simulink model "test1"  (R2020a)
settings: Solver=VariableStepAuto  StartTime=0.0  StopTime=inf  FixedStep=Ts  RelTol=1e-3
PostLoadFcn:
  | , if any(exist('dsrtsu_mdlpostloadfcn', 'file') ~= 0), dsrtsu_mdlpostloadfcn('Execute', bdroot); end,
InitFcn:
  | , if any(exist('rtifpga_mdlclblib', 'file') ~= 0), rtifpga_mdlclblib('Init', bdroot); end,
model workspace (MAT data in the model file):
  FPGA_test1_1_Interrupt_1_1_write = Simulink.Signal
  FPGA_test1_1_Interrupt_1_1_write.Description = 'RTIFPGA'
  FPGA_test1_1_Interrupt_1_1_write.DataType = 'double'
  FPGA_test1_1_Interrupt_1_1_write.Dimensions = '1'
  FPGA_test1_1_Interrupt_1_1_write.DimensionsMode = 'auto'
  FPGA_test1_1_Interrupt_1_1_write.Complexity = 'auto'
  FPGA_test1_1_Interrupt_1_1_write.SampleTime = -1
  FPGA_test1_1_Interrupt_1_1_write.SamplingMode = 'auto'
  FPGA_test1_1_Register_1_1_1_write = Simulink.Signal
  FPGA_test1_1_Register_1_1_1_write.Description = 'RTIFPGA'
  FPGA_test1_1_Register_1_1_1_write.DataType = 'double'
  FPGA_test1_1_Register_1_1_1_write.Dimensions = '1'
  FPGA_test1_1_Register_1_1_1_write.DimensionsMode = 'auto'
  FPGA_test1_1_Register_1_1_1_write.Complexity = 'auto'
  FPGA_test1_1_Register_1_1_1_write.SampleTime = -1
  FPGA_test1_1_Register_1_1_1_write.SamplingMode = 'auto'
  FPGA_test1_1_Register_2_1_1_write = Simulink.Signal
  FPGA_test1_1_Register_2_1_1_write.Description = 'RTIFPGA'
  FPGA_test1_1_Register_2_1_1_write.DataType = 'double'
  FPGA_test1_1_Register_2_1_1_write.Dimensions = '1'
  FPGA_test1_1_Register_2_1_1_write.DimensionsMode = 'auto'
  FPGA_test1_1_Register_2_1_1_write.Complexity = 'auto'
  FPGA_test1_1_Register_2_1_1_write.SampleTime = -1
  FPGA_test1_1_Register_2_1_1_write.SamplingMode = 'auto'
  FPGA_test1_1_Register_3_1_1_write = Simulink.Signal
  FPGA_test1_1_Register_3_1_1_write.Description = 'RTIFPGA'
  FPGA_test1_1_Register_3_1_1_write.DataType = 'double'
  FPGA_test1_1_Register_3_1_1_write.Dimensions = '1'
  FPGA_test1_1_Register_3_1_1_write.DimensionsMode = 'auto'
  FPGA_test1_1_Register_3_1_1_write.Complexity = 'auto'
  FPGA_test1_1_Register_3_1_1_write.SampleTime = -1
  FPGA_test1_1_Register_3_1_1_write.SamplingMode = 'auto'
  FPGA_test1_1_Register_4_1_1_write = Simulink.Signal
  FPGA_test1_1_Register_4_1_1_write.Description = 'RTIFPGA'
  FPGA_test1_1_Register_4_1_1_write.DataType = 'double'
  FPGA_test1_1_Register_4_1_1_write.Dimensions = '1'
  FPGA_test1_1_Register_4_1_1_write.DimensionsMode = 'auto'
  FPGA_test1_1_Register_4_1_1_write.Complexity = 'auto'
  FPGA_test1_1_Register_4_1_1_write.SampleTime = -1
  FPGA_test1_1_Register_4_1_1_write.SamplingMode = 'auto'
values from neighbouring files (symbols this model uses):
  clamp_threshold = 200    [param.m]
  io_fixed_gain = 10*1000/(3*100)    (= 33.3333333333)    [param.m]
  io_sonda_gain = 10/0.010    (= 1000)    [param.m]
  ioa_gain = 1    [param.m]
  ioa_offset = 0.12    [param.m]
  iob_gain = 1    [param.m]
  iob_offset = 0.06    [param.m]
  ioc_gain = 1    [param.m]
  ioc_offset = -0.1    [param.m]
  Ts = 20e-6    (= 2e-05)    [param.m]
  vclamp_gain = 1010    [param.m]
  vclamp_offset = 10.5    [param.m]
  vi_fixed_gain = 10*44    (= 440)    [param.m]
  vi_sonda_gain = 10*200    (= 2000)    [param.m]
  via_gain = 1    [param.m]
  via_offset = 2.2    [param.m]
  vib_gain = 1    [param.m]
  vib_offset = 3    [param.m]
  vic_gain = 1    [param.m]
  vic_offset = 4.2    [param.m]
libraries: xbsIndex_r4 x428, rti1202lib_adc_class1 x9, rtiproclib x6, simulink x2, rtifpgainterfacelib x1
(part 1 of 7)
Description:
  | Standard RTI1202 template.
  | Supported MATLAB version:  R2020a.
settings Model: Tag=RTI1202  DSRTSU_INTERNAL_RTI_VER=570  DSRTSU_INTERNAL_RTI_TYPE=rti1202  RTICANMMDATA=struct('GeneralSetupData',struct('modelroot','D:\MarcosGomez\test1','generalsettings',struct('filesettings',struct('destfolder',struct('Name','RTICANMM_FILES','Check',1),'buildfolder',struct('Name','.','Check',1),'AbsDestfolder',struct('Name','D:\MarcosGomez\test1\RTICANMM_FILES'),'AbsBuildfolder',struct('Name','D:\MarcosGomez\test1'))),'options',struct('addpaths',1,'rmpaths',1,'addtrcexclusion',true,'cannavigator',struct('checkmonitoring',0),'show_usrtrc',0,'use_usrtrc',0),'advanced',struct('options',ones(1,100)),'MPSetup',{{}},'RTI',struct('Type','RTI1202','Ver','7.15','Date','02-Nov-2020'),'modelname','test1','block','test1'))  DSRTSU_INTERNAL_RTIFPGA=170  OrderedModelArguments=off  Creator=dSPACE2020b  LastModifiedBy=dspace
settings DataIOCC: ReturnWorkspaceOutputs=off
settings OptimizationCC: BlockReduction=off  OptimizeBlockIOStorage=off  BufferReuse=off  GlobalBufferReuse=off  ExpressionFolding=off  LocalBlockOutputs=off  OptimizeDataStoreBuffers=off  BusAssignmentInplaceUpdate=off
settings DebuggingCC: PregeneratedLibrarySubsystemCodeDiagnostic=none  ArithmeticOperatorsInVariantConditions=warning
settings HardwareCC: ProdBitPerPointer=32  ProdBitPerSizeT=32  ProdBitPerPtrDiffT=32  ProdLargestAtomicInteger=Integer  ProdEndianess=BigEndian  ProdWordSize=32  ProdLongLongMode=on  ProdHWDeviceType=Custom Processor->Custom  TargetIntDivRoundTo=Zero  TargetEndianess=BigEndian  TargetHWDeviceType=Custom Processor->Custom
settings ModelReferenceCC: EnableParallelModelReferenceBuilds=on  ParallelModelReferenceMATLABWorkerInit=Load Top Model
settings SFSimCC: SimUseLocalCustomCode=off  MATLABDynamicMemAlloc=off  CustomCodeUndefinedFunction=UseInterfaceOnly
settings RTWCC: Description=dSPACE DS1202 Hardware Platform  SystemTargetFile=rti1202.tlc  MakeCommand=make_rti  TemplateMakefile=rti1202.tmf  RTWUseLocalCustomCode=off
settings CodeAppCC: StateflowObjectComments=on
settings STFCustomTargetCC: ParMdlRefBuildCompliant=on  SystemTargetFile=rti1202.tlc
settings GRTTargetCC: TargetLangStandard=C89/C90 (ANSI)  CompOptLevelCompliant=off  ConcurrentExecutionCompliant=off  CombineOutputUpdateFcns=off  MatFileLogging=off  CPPClassGenCompliant=off  UseToolchainInfoCompliant=off
settings ConfigComp: CovMetricSettings=dswe

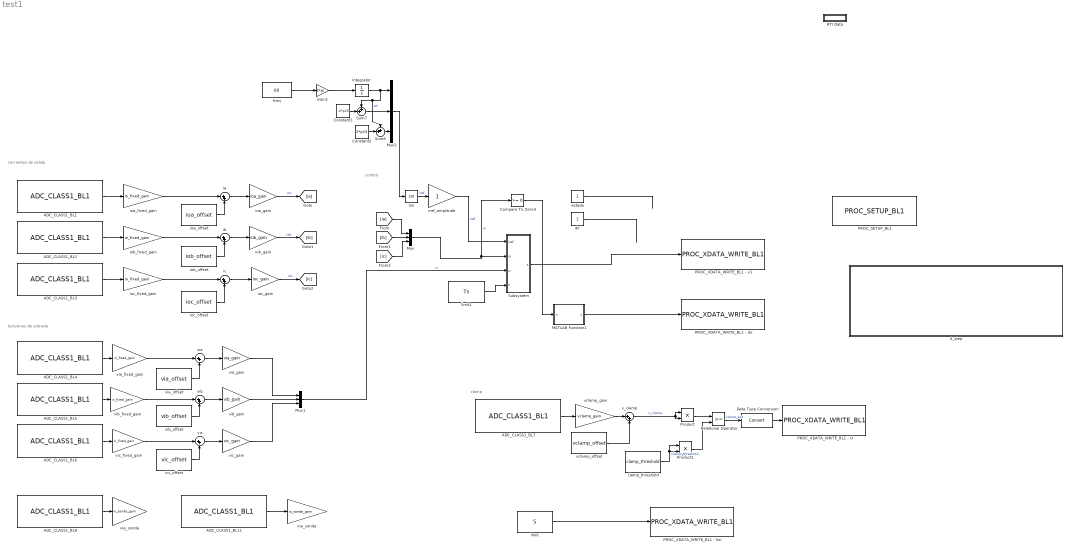
== system test1 ==
  note: control
  note: clamp
  note: tensiones de entrada
  note: corrientes de salida
  4_step : Subsystem
  ADC_CLASS1_BL1 : rti1202lib_adc_class1/ADC_CLASS1_BL1  DSProperties=struct('RTI',struct('Version',uint32(1),'BlockType',struct('isSLSource',uint8(1),'isSLSink',uint8(1),'isHWSource',uint8(0),'isHWSink',uint8(1),'isSetup',uint8(0),'isInline',uint8(1),'isNonInline',uint8(0),'isInterrupt',uint8(0),'isChannelwise',uint8(1)),'IOBoardType',{{'DS120X','STD','ADCC1'}},'UnitType','ADC','Identifier','ADC','DialogType','ML','BlockSet','NONE','SlaveProcessor','NONE'))  RTIBlockInterface=struct('InputPortsActive',0,'InputPortsWidth',int32(1),'InputPortsDataType',{{'SS_BOOLEAN'}},'InputPortsName',{{'Continue'}},'OutputPortsActive',[1 0],'OutputPortsWidth',int32([1 1]),'OutputPortsDataType',{{'SS_DOUBLE','SS_INT16'}},'OutputPortsName',{{'ADC','Status'}},'DialogFcn','rti120xstdadcc1adcgui','SampleTime',{{-1}},'InitLevel',3,'IconTransparency','on','BlockDisplay',{{['ADC CL1\nChannel: 1'],'center'}},'BlockName',struct('Token',{{'ADC_CLASS1_BL1'}}))  RTIBlockParameters=struct('ReadMode',{{1,'OFF',[1 2]}},'ChannelNo',{{1,'OFF',[]}},'ConversionMode',{{1,'OFF',[1 2]}},'TriggerSource',{{1,'OFF',[1 2]}},'TriggerLineIn',{{1,'OFF',[1 16]}},'SampleMode',{{1,'OFF',[1 2]}},'BurstTriggerSource',{{1,'OFF',[1 2]}},'BurstTriggerLine',{{1,'OFF',[1 16]}},'ConvTriggerSource',{{3,'OFF',[1 3]}},'ConvTriggerLine',{{1,'OFF',[1 16]}},'ConvPeriod',{{'100e-6','OFF',[1e-6 1.34]}},'ConvPeriodCheck',{{0,'OFF',[]}},'BurstSize',{{'10','OFF',[]}},'BurstSizeCheck',{{0,'OFF',[]}},'DataSetOffset',{{'0','OFF',[]}},'DataSetOffsetCheck',{{0,'OFF',[]}},'DataSetLength',{{'1','OFF',[]}},'DataSetLengthCheck',{{0,'OFF',[]}},'EnableTriggerEvent',{{0,'OFF',[0 1]}},'TriggerMode',{{2,'OFF',[1 3]}},'TriggerLineOut',{{1,'OFF',[1 16]}},'ADCSWStartEnable',{{0,'OFF',[0 1]}},'SampleTime',{{'-1','OFF',[-1 inf]}},'SampleTimeCheck',{{1,'OFF',[]}},'StatusPortEnable',{{0,'OFF',[0 1]}},'TLCFileName',{{'rti120xadc_c1_adc','OFF',[]}})  RTISFcnParameters=struct('ReadMode','int16','ChannelNo','int16','ConversionMode','int16','TriggerSource','int16','TriggerLineIn','int16','SampleMode','int16','BurstTriggerSource','int16','BurstTriggerLine','int16','ConvTriggerSource','int16','ConvTriggerLine','int16','ConvPeriod','double','BurstSize','int16','DataSetOffset','int16','DataSetLength','int16','EnableTriggerEvent','int16','TriggerMode','int16','TriggerLineOut','int16','ADCSWStartEnable','int16','SampleTime','double','StatusPortEnable','int16','TLCFileName','char')  RTIBlockParaDefault=struct('ReadMode',1,'ChannelNo',1,'ConversionMode',1,'TriggerSource',1,'TriggerLineIn',1,'SampleMode',1,'BurstTriggerSource',1,'BurstTriggerLine',1,'ConvTriggerSource',3,'ConvTriggerLine',1,'ConvPeriod',0.0001,'ConvPeriodCheck',0,'BurstSize',10,'BurstSizeCheck',0,'DataSetOffset',0,'DataSetOffsetCheck',0,'DataSetLength',1,'DataSetLengthCheck',0,'EnableTriggerEvent',0,'TriggerMode',2,'TriggerLineOut',1,'ADCSWStartEnable',0,'SampleTime',-1,'SampleTimeCheck',1,'StatusPortEnable',0,'TLCFileName','rti120xadc_c1_adc')
  ADC_CLASS1_BL11 : rti1202lib_adc_class1/ADC_CLASS1_BL1  DSProperties=struct('RTI',struct('Version',uint32(1),'BlockType',struct('isSLSource',uint8(1),'isSLSink',uint8(1),'isHWSource',uint8(0),'isHWSink',uint8(1),'isSetup',uint8(0),'isInline',uint8(1),'isNonInline',uint8(0),'isInterrupt',uint8(0),'isChannelwise',uint8(1)),'IOBoardType',{{'DS120X','STD','ADCC1'}},'UnitType','ADC','Identifier','ADC','DialogType','ML','BlockSet','NONE','SlaveProcessor','NONE'))  RTIBlockInterface=struct('InputPortsActive',0,'InputPortsWidth',int32(1),'InputPortsDataType',{{'SS_BOOLEAN'}},'InputPortsName',{{'Continue'}},'OutputPortsActive',[1 0],'OutputPortsWidth',int32([1 1]),'OutputPortsDataType',{{'SS_DOUBLE','SS_INT16'}},'OutputPortsName',{{'ADC','Status'}},'DialogFcn','rti120xstdadcc1adcgui','SampleTime',{{-1}},'InitLevel',3,'IconTransparency','on','BlockDisplay',{{['ADC CL1\nChannel: 16'],'center'}},'BlockName',struct('Token',{{'ADC_CLASS1_BL1'}}))  RTIBlockParameters=struct('ReadMode',{{1,'OFF',[1 2]}},'ChannelNo',{{16,'OFF',[]}},'ConversionMode',{{1,'OFF',[1 2]}},'TriggerSource',{{1,'OFF',[1 2]}},'TriggerLineIn',{{1,'OFF',[1 16]}},'SampleMode',{{1,'OFF',[1 2]}},'BurstTriggerSource',{{1,'OFF',[1 2]}},'BurstTriggerLine',{{1,'OFF',[1 16]}},'ConvTriggerSource',{{3,'OFF',[1 3]}},'ConvTriggerLine',{{1,'OFF',[1 16]}},'ConvPeriod',{{'100e-6','OFF',[1e-6 1.34]}},'ConvPeriodCheck',{{0,'OFF',[]}},'BurstSize',{{'10','OFF',[]}},'BurstSizeCheck',{{0,'OFF',[]}},'DataSetOffset',{{'0','OFF',[]}},'DataSetOffsetCheck',{{0,'OFF',[]}},'DataSetLength',{{'1','OFF',[]}},'DataSetLengthCheck',{{0,'OFF',[]}},'EnableTriggerEvent',{{0,'OFF',[0 1]}},'TriggerMode',{{2,'OFF',[1 3]}},'TriggerLineOut',{{1,'OFF',[1 16]}},'ADCSWStartEnable',{{0,'OFF',[0 1]}},'SampleTime',{{'-1','OFF',[-1 inf]}},'SampleTimeCheck',{{1,'OFF',[]}},'StatusPortEnable',{{0,'OFF',[0 1]}},'TLCFileName',{{'rti120xadc_c1_adc','OFF',[]}})  RTISFcnParameters=struct('ReadMode','int16','ChannelNo','int16','ConversionMode','int16','TriggerSource','int16','TriggerLineIn','int16','SampleMode','int16','BurstTriggerSource','int16','BurstTriggerLine','int16','ConvTriggerSource','int16','ConvTriggerLine','int16','ConvPeriod','double','BurstSize','int16','DataSetOffset','int16','DataSetLength','int16','EnableTriggerEvent','int16','TriggerMode','int16','TriggerLineOut','int16','ADCSWStartEnable','int16','SampleTime','double','StatusPortEnable','int16','TLCFileName','char')  RTIBlockParaDefault=struct('ReadMode',1,'ChannelNo',1,'ConversionMode',1,'TriggerSource',1,'TriggerLineIn',1,'SampleMode',1,'BurstTriggerSource',1,'BurstTriggerLine',1,'ConvTriggerSource',3,'ConvTriggerLine',1,'ConvPeriod',0.0001,'ConvPeriodCheck',0,'BurstSize',10,'BurstSizeCheck',0,'DataSetOffset',0,'DataSetOffsetCheck',0,'DataSetLength',1,'DataSetLengthCheck',0,'EnableTriggerEvent',0,'TriggerMode',2,'TriggerLineOut',1,'ADCSWStartEnable',0,'SampleTime',-1,'SampleTimeCheck',1,'StatusPortEnable',0,'TLCFileName','rti120xadc_c1_adc')
  ADC_CLASS1_BL2 : rti1202lib_adc_class1/ADC_CLASS1_BL1  DSProperties=struct('RTI',struct('Version',uint32(1),'BlockType',struct('isSLSource',uint8(1),'isSLSink',uint8(1),'isHWSource',uint8(0),'isHWSink',uint8(1),'isSetup',uint8(0),'isInline',uint8(1),'isNonInline',uint8(0),'isInterrupt',uint8(0),'isChannelwise',uint8(1)),'IOBoardType',{{'DS120X','STD','ADCC1'}},'UnitType','ADC','Identifier','ADC','DialogType','ML','BlockSet','NONE','SlaveProcessor','NONE'))  RTIBlockInterface=struct('InputPortsActive',0,'InputPortsWidth',int32(1),'InputPortsDataType',{{'SS_BOOLEAN'}},'InputPortsName',{{'Continue'}},'OutputPortsActive',[1 0],'OutputPortsWidth',int32([1 1]),'OutputPortsDataType',{{'SS_DOUBLE','SS_INT16'}},'OutputPortsName',{{'ADC','Status'}},'DialogFcn','rti120xstdadcc1adcgui','SampleTime',{{-1}},'InitLevel',3,'IconTransparency','on','BlockDisplay',{{['ADC CL1\nChannel: 2'],'center'}},'BlockName',struct('Token',{{'ADC_CLASS1_BL1'}}))  RTIBlockParameters=struct('ReadMode',{{1,'OFF',[1 2]}},'ChannelNo',{{2,'OFF',[]}},'ConversionMode',{{1,'OFF',[1 2]}},'TriggerSource',{{1,'OFF',[1 2]}},'TriggerLineIn',{{1,'OFF',[1 16]}},'SampleMode',{{1,'OFF',[1 2]}},'BurstTriggerSource',{{1,'OFF',[1 2]}},'BurstTriggerLine',{{1,'OFF',[1 16]}},'ConvTriggerSource',{{3,'OFF',[1 3]}},'ConvTriggerLine',{{1,'OFF',[1 16]}},'ConvPeriod',{{'100e-6','OFF',[1e-6 1.34]}},'ConvPeriodCheck',{{0,'OFF',[]}},'BurstSize',{{'10','OFF',[]}},'BurstSizeCheck',{{0,'OFF',[]}},'DataSetOffset',{{'0','OFF',[]}},'DataSetOffsetCheck',{{0,'OFF',[]}},'DataSetLength',{{'1','OFF',[]}},'DataSetLengthCheck',{{0,'OFF',[]}},'EnableTriggerEvent',{{0,'OFF',[0 1]}},'TriggerMode',{{2,'OFF',[1 3]}},'TriggerLineOut',{{1,'OFF',[1 16]}},'ADCSWStartEnable',{{0,'OFF',[0 1]}},'SampleTime',{{'-1','OFF',[-1 inf]}},'SampleTimeCheck',{{1,'OFF',[]}},'StatusPortEnable',{{0,'OFF',[0 1]}},'TLCFileName',{{'rti120xadc_c1_adc','OFF',[]}})  RTISFcnParameters=struct('ReadMode','int16','ChannelNo','int16','ConversionMode','int16','TriggerSource','int16','TriggerLineIn','int16','SampleMode','int16','BurstTriggerSource','int16','BurstTriggerLine','int16','ConvTriggerSource','int16','ConvTriggerLine','int16','ConvPeriod','double','BurstSize','int16','DataSetOffset','int16','DataSetLength','int16','EnableTriggerEvent','int16','TriggerMode','int16','TriggerLineOut','int16','ADCSWStartEnable','int16','SampleTime','double','StatusPortEnable','int16','TLCFileName','char')  RTIBlockParaDefault=struct('ReadMode',1,'ChannelNo',1,'ConversionMode',1,'TriggerSource',1,'TriggerLineIn',1,'SampleMode',1,'BurstTriggerSource',1,'BurstTriggerLine',1,'ConvTriggerSource',3,'ConvTriggerLine',1,'ConvPeriod',0.0001,'ConvPeriodCheck',0,'BurstSize',10,'BurstSizeCheck',0,'DataSetOffset',0,'DataSetOffsetCheck',0,'DataSetLength',1,'DataSetLengthCheck',0,'EnableTriggerEvent',0,'TriggerMode',2,'TriggerLineOut',1,'ADCSWStartEnable',0,'SampleTime',-1,'SampleTimeCheck',1,'StatusPortEnable',0,'TLCFileName','rti120xadc_c1_adc')
  ADC_CLASS1_BL3 : rti1202lib_adc_class1/ADC_CLASS1_BL1  DSProperties=struct('RTI',struct('Version',uint32(1),'BlockType',struct('isSLSource',uint8(1),'isSLSink',uint8(1),'isHWSource',uint8(0),'isHWSink',uint8(1),'isSetup',uint8(0),'isInline',uint8(1),'isNonInline',uint8(0),'isInterrupt',uint8(0),'isChannelwise',uint8(1)),'IOBoardType',{{'DS120X','STD','ADCC1'}},'UnitType','ADC','Identifier','ADC','DialogType','ML','BlockSet','NONE','SlaveProcessor','NONE'))  RTIBlockInterface=struct('InputPortsActive',0,'InputPortsWidth',int32(1),'InputPortsDataType',{{'SS_BOOLEAN'}},'InputPortsName',{{'Continue'}},'OutputPortsActive',[1 0],'OutputPortsWidth',int32([1 1]),'OutputPortsDataType',{{'SS_DOUBLE','SS_INT16'}},'OutputPortsName',{{'ADC','Status'}},'DialogFcn','rti120xstdadcc1adcgui','SampleTime',{{-1}},'InitLevel',3,'IconTransparency','on','BlockDisplay',{{['ADC CL1\nChannel: 3'],'center'}},'BlockName',struct('Token',{{'ADC_CLASS1_BL1'}}))  RTIBlockParameters=struct('ReadMode',{{1,'OFF',[1 2]}},'ChannelNo',{{3,'OFF',[]}},'ConversionMode',{{1,'OFF',[1 2]}},'TriggerSource',{{1,'OFF',[1 2]}},'TriggerLineIn',{{1,'OFF',[1 16]}},'SampleMode',{{1,'OFF',[1 2]}},'BurstTriggerSource',{{1,'OFF',[1 2]}},'BurstTriggerLine',{{1,'OFF',[1 16]}},'ConvTriggerSource',{{3,'OFF',[1 3]}},'ConvTriggerLine',{{1,'OFF',[1 16]}},'ConvPeriod',{{'100e-6','OFF',[1e-6 1.34]}},'ConvPeriodCheck',{{0,'OFF',[]}},'BurstSize',{{'10','OFF',[]}},'BurstSizeCheck',{{0,'OFF',[]}},'DataSetOffset',{{'0','OFF',[]}},'DataSetOffsetCheck',{{0,'OFF',[]}},'DataSetLength',{{'1','OFF',[]}},'DataSetLengthCheck',{{0,'OFF',[]}},'EnableTriggerEvent',{{0,'OFF',[0 1]}},'TriggerMode',{{2,'OFF',[1 3]}},'TriggerLineOut',{{1,'OFF',[1 16]}},'ADCSWStartEnable',{{0,'OFF',[0 1]}},'SampleTime',{{'-1','OFF',[-1 inf]}},'SampleTimeCheck',{{1,'OFF',[]}},'StatusPortEnable',{{0,'OFF',[0 1]}},'TLCFileName',{{'rti120xadc_c1_adc','OFF',[]}})  RTISFcnParameters=struct('ReadMode','int16','ChannelNo','int16','ConversionMode','int16','TriggerSource','int16','TriggerLineIn','int16','SampleMode','int16','BurstTriggerSource','int16','BurstTriggerLine','int16','ConvTriggerSource','int16','ConvTriggerLine','int16','ConvPeriod','double','BurstSize','int16','DataSetOffset','int16','DataSetLength','int16','EnableTriggerEvent','int16','TriggerMode','int16','TriggerLineOut','int16','ADCSWStartEnable','int16','SampleTime','double','StatusPortEnable','int16','TLCFileName','char')  RTIBlockParaDefault=struct('ReadMode',1,'ChannelNo',1,'ConversionMode',1,'TriggerSource',1,'TriggerLineIn',1,'SampleMode',1,'BurstTriggerSource',1,'BurstTriggerLine',1,'ConvTriggerSource',3,'ConvTriggerLine',1,'ConvPeriod',0.0001,'ConvPeriodCheck',0,'BurstSize',10,'BurstSizeCheck',0,'DataSetOffset',0,'DataSetOffsetCheck',0,'DataSetLength',1,'DataSetLengthCheck',0,'EnableTriggerEvent',0,'TriggerMode',2,'TriggerLineOut',1,'ADCSWStartEnable',0,'SampleTime',-1,'SampleTimeCheck',1,'StatusPortEnable',0,'TLCFileName','rti120xadc_c1_adc')
  ADC_CLASS1_BL4 : rti1202lib_adc_class1/ADC_CLASS1_BL1  DSProperties=struct('RTI',struct('Version',uint32(1),'BlockType',struct('isSLSource',uint8(1),'isSLSink',uint8(1),'isHWSource',uint8(0),'isHWSink',uint8(1),'isSetup',uint8(0),'isInline',uint8(1),'isNonInline',uint8(0),'isInterrupt',uint8(0),'isChannelwise',uint8(1)),'IOBoardType',{{'DS120X','STD','ADCC1'}},'UnitType','ADC','Identifier','ADC','DialogType','ML','BlockSet','NONE','SlaveProcessor','NONE'))  RTIBlockInterface=struct('InputPortsActive',0,'InputPortsWidth',int32(1),'InputPortsDataType',{{'SS_BOOLEAN'}},'InputPortsName',{{'Continue'}},'OutputPortsActive',[1 0],'OutputPortsWidth',int32([1 1]),'OutputPortsDataType',{{'SS_DOUBLE','SS_INT16'}},'OutputPortsName',{{'ADC','Status'}},'DialogFcn','rti120xstdadcc1adcgui','SampleTime',{{-1}},'InitLevel',3,'IconTransparency','on','BlockDisplay',{{['ADC CL1\nChannel: 4'],'center'}},'BlockName',struct('Token',{{'ADC_CLASS1_BL1'}}))  RTIBlockParameters=struct('ReadMode',{{1,'OFF',[1 2]}},'ChannelNo',{{4,'OFF',[]}},'ConversionMode',{{1,'OFF',[1 2]}},'TriggerSource',{{1,'OFF',[1 2]}},'TriggerLineIn',{{1,'OFF',[1 16]}},'SampleMode',{{1,'OFF',[1 2]}},'BurstTriggerSource',{{1,'OFF',[1 2]}},'BurstTriggerLine',{{1,'OFF',[1 16]}},'ConvTriggerSource',{{3,'OFF',[1 3]}},'ConvTriggerLine',{{1,'OFF',[1 16]}},'ConvPeriod',{{'100e-6','OFF',[1e-6 1.34]}},'ConvPeriodCheck',{{0,'OFF',[]}},'BurstSize',{{'10','OFF',[]}},'BurstSizeCheck',{{0,'OFF',[]}},'DataSetOffset',{{'0','OFF',[]}},'DataSetOffsetCheck',{{0,'OFF',[]}},'DataSetLength',{{'1','OFF',[]}},'DataSetLengthCheck',{{0,'OFF',[]}},'EnableTriggerEvent',{{0,'OFF',[0 1]}},'TriggerMode',{{2,'OFF',[1 3]}},'TriggerLineOut',{{1,'OFF',[1 16]}},'ADCSWStartEnable',{{0,'OFF',[0 1]}},'SampleTime',{{'-1','OFF',[-1 inf]}},'SampleTimeCheck',{{1,'OFF',[]}},'StatusPortEnable',{{0,'OFF',[0 1]}},'TLCFileName',{{'rti120xadc_c1_adc','OFF',[]}})  RTISFcnParameters=struct('ReadMode','int16','ChannelNo','int16','ConversionMode','int16','TriggerSource','int16','TriggerLineIn','int16','SampleMode','int16','BurstTriggerSource','int16','BurstTriggerLine','int16','ConvTriggerSource','int16','ConvTriggerLine','int16','ConvPeriod','double','BurstSize','int16','DataSetOffset','int16','DataSetLength','int16','EnableTriggerEvent','int16','TriggerMode','int16','TriggerLineOut','int16','ADCSWStartEnable','int16','SampleTime','double','StatusPortEnable','int16','TLCFileName','char')  RTIBlockParaDefault=struct('ReadMode',1,'ChannelNo',1,'ConversionMode',1,'TriggerSource',1,'TriggerLineIn',1,'SampleMode',1,'BurstTriggerSource',1,'BurstTriggerLine',1,'ConvTriggerSource',3,'ConvTriggerLine',1,'ConvPeriod',0.0001,'ConvPeriodCheck',0,'BurstSize',10,'BurstSizeCheck',0,'DataSetOffset',0,'DataSetOffsetCheck',0,'DataSetLength',1,'DataSetLengthCheck',0,'EnableTriggerEvent',0,'TriggerMode',2,'TriggerLineOut',1,'ADCSWStartEnable',0,'SampleTime',-1,'SampleTimeCheck',1,'StatusPortEnable',0,'TLCFileName','rti120xadc_c1_adc')
  ADC_CLASS1_BL5 : rti1202lib_adc_class1/ADC_CLASS1_BL1  DSProperties=struct('RTI',struct('Version',uint32(1),'BlockType',struct('isSLSource',uint8(1),'isSLSink',uint8(1),'isHWSource',uint8(0),'isHWSink',uint8(1),'isSetup',uint8(0),'isInline',uint8(1),'isNonInline',uint8(0),'isInterrupt',uint8(0),'isChannelwise',uint8(1)),'IOBoardType',{{'DS120X','STD','ADCC1'}},'UnitType','ADC','Identifier','ADC','DialogType','ML','BlockSet','NONE','SlaveProcessor','NONE'))  RTIBlockInterface=struct('InputPortsActive',0,'InputPortsWidth',int32(1),'InputPortsDataType',{{'SS_BOOLEAN'}},'InputPortsName',{{'Continue'}},'OutputPortsActive',[1 0],'OutputPortsWidth',int32([1 1]),'OutputPortsDataType',{{'SS_DOUBLE','SS_INT16'}},'OutputPortsName',{{'ADC','Status'}},'DialogFcn','rti120xstdadcc1adcgui','SampleTime',{{-1}},'InitLevel',3,'IconTransparency','on','BlockDisplay',{{['ADC CL1\nChannel: 5'],'center'}},'BlockName',struct('Token',{{'ADC_CLASS1_BL1'}}))  RTIBlockParameters=struct('ReadMode',{{1,'OFF',[1 2]}},'ChannelNo',{{5,'OFF',[]}},'ConversionMode',{{1,'OFF',[1 2]}},'TriggerSource',{{1,'OFF',[1 2]}},'TriggerLineIn',{{1,'OFF',[1 16]}},'SampleMode',{{1,'OFF',[1 2]}},'BurstTriggerSource',{{1,'OFF',[1 2]}},'BurstTriggerLine',{{1,'OFF',[1 16]}},'ConvTriggerSource',{{3,'OFF',[1 3]}},'ConvTriggerLine',{{1,'OFF',[1 16]}},'ConvPeriod',{{'100e-6','OFF',[1e-6 1.34]}},'ConvPeriodCheck',{{0,'OFF',[]}},'BurstSize',{{'10','OFF',[]}},'BurstSizeCheck',{{0,'OFF',[]}},'DataSetOffset',{{'0','OFF',[]}},'DataSetOffsetCheck',{{0,'OFF',[]}},'DataSetLength',{{'1','OFF',[]}},'DataSetLengthCheck',{{0,'OFF',[]}},'EnableTriggerEvent',{{0,'OFF',[0 1]}},'TriggerMode',{{2,'OFF',[1 3]}},'TriggerLineOut',{{1,'OFF',[1 16]}},'ADCSWStartEnable',{{0,'OFF',[0 1]}},'SampleTime',{{'-1','OFF',[-1 inf]}},'SampleTimeCheck',{{1,'OFF',[]}},'StatusPortEnable',{{0,'OFF',[0 1]}},'TLCFileName',{{'rti120xadc_c1_adc','OFF',[]}})  RTISFcnParameters=struct('ReadMode','int16','ChannelNo','int16','ConversionMode','int16','TriggerSource','int16','TriggerLineIn','int16','SampleMode','int16','BurstTriggerSource','int16','BurstTriggerLine','int16','ConvTriggerSource','int16','ConvTriggerLine','int16','ConvPeriod','double','BurstSize','int16','DataSetOffset','int16','DataSetLength','int16','EnableTriggerEvent','int16','TriggerMode','int16','TriggerLineOut','int16','ADCSWStartEnable','int16','SampleTime','double','StatusPortEnable','int16','TLCFileName','char')  RTIBlockParaDefault=struct('ReadMode',1,'ChannelNo',1,'ConversionMode',1,'TriggerSource',1,'TriggerLineIn',1,'SampleMode',1,'BurstTriggerSource',1,'BurstTriggerLine',1,'ConvTriggerSource',3,'ConvTriggerLine',1,'ConvPeriod',0.0001,'ConvPeriodCheck',0,'BurstSize',10,'BurstSizeCheck',0,'DataSetOffset',0,'DataSetOffsetCheck',0,'DataSetLength',1,'DataSetLengthCheck',0,'EnableTriggerEvent',0,'TriggerMode',2,'TriggerLineOut',1,'ADCSWStartEnable',0,'SampleTime',-1,'SampleTimeCheck',1,'StatusPortEnable',0,'TLCFileName','rti120xadc_c1_adc')
  ADC_CLASS1_BL6 : rti1202lib_adc_class1/ADC_CLASS1_BL1  DSProperties=struct('RTI',struct('Version',uint32(1),'BlockType',struct('isSLSource',uint8(1),'isSLSink',uint8(1),'isHWSource',uint8(0),'isHWSink',uint8(1),'isSetup',uint8(0),'isInline',uint8(1),'isNonInline',uint8(0),'isInterrupt',uint8(0),'isChannelwise',uint8(1)),'IOBoardType',{{'DS120X','STD','ADCC1'}},'UnitType','ADC','Identifier','ADC','DialogType','ML','BlockSet','NONE','SlaveProcessor','NONE'))  RTIBlockInterface=struct('InputPortsActive',0,'InputPortsWidth',int32(1),'InputPortsDataType',{{'SS_BOOLEAN'}},'InputPortsName',{{'Continue'}},'OutputPortsActive',[1 0],'OutputPortsWidth',int32([1 1]),'OutputPortsDataType',{{'SS_DOUBLE','SS_INT16'}},'OutputPortsName',{{'ADC','Status'}},'DialogFcn','rti120xstdadcc1adcgui','SampleTime',{{-1}},'InitLevel',3,'IconTransparency','on','BlockDisplay',{{['ADC CL1\nChannel: 6'],'center'}},'BlockName',struct('Token',{{'ADC_CLASS1_BL1'}}))  RTIBlockParameters=struct('ReadMode',{{1,'OFF',[1 2]}},'ChannelNo',{{6,'OFF',[]}},'ConversionMode',{{1,'OFF',[1 2]}},'TriggerSource',{{1,'OFF',[1 2]}},'TriggerLineIn',{{1,'OFF',[1 16]}},'SampleMode',{{1,'OFF',[1 2]}},'BurstTriggerSource',{{1,'OFF',[1 2]}},'BurstTriggerLine',{{1,'OFF',[1 16]}},'ConvTriggerSource',{{3,'OFF',[1 3]}},'ConvTriggerLine',{{1,'OFF',[1 16]}},'ConvPeriod',{{'100e-6','OFF',[1e-6 1.34]}},'ConvPeriodCheck',{{0,'OFF',[]}},'BurstSize',{{'10','OFF',[]}},'BurstSizeCheck',{{0,'OFF',[]}},'DataSetOffset',{{'0','OFF',[]}},'DataSetOffsetCheck',{{0,'OFF',[]}},'DataSetLength',{{'1','OFF',[]}},'DataSetLengthCheck',{{0,'OFF',[]}},'EnableTriggerEvent',{{0,'OFF',[0 1]}},'TriggerMode',{{2,'OFF',[1 3]}},'TriggerLineOut',{{1,'OFF',[1 16]}},'ADCSWStartEnable',{{0,'OFF',[0 1]}},'SampleTime',{{'-1','OFF',[-1 inf]}},'SampleTimeCheck',{{1,'OFF',[]}},'StatusPortEnable',{{0,'OFF',[0 1]}},'TLCFileName',{{'rti120xadc_c1_adc','OFF',[]}})  RTISFcnParameters=struct('ReadMode','int16','ChannelNo','int16','ConversionMode','int16','TriggerSource','int16','TriggerLineIn','int16','SampleMode','int16','BurstTriggerSource','int16','BurstTriggerLine','int16','ConvTriggerSource','int16','ConvTriggerLine','int16','ConvPeriod','double','BurstSize','int16','DataSetOffset','int16','DataSetLength','int16','EnableTriggerEvent','int16','TriggerMode','int16','TriggerLineOut','int16','ADCSWStartEnable','int16','SampleTime','double','StatusPortEnable','int16','TLCFileName','char')  RTIBlockParaDefault=struct('ReadMode',1,'ChannelNo',1,'ConversionMode',1,'TriggerSource',1,'TriggerLineIn',1,'SampleMode',1,'BurstTriggerSource',1,'BurstTriggerLine',1,'ConvTriggerSource',3,'ConvTriggerLine',1,'ConvPeriod',0.0001,'ConvPeriodCheck',0,'BurstSize',10,'BurstSizeCheck',0,'DataSetOffset',0,'DataSetOffsetCheck',0,'DataSetLength',1,'DataSetLengthCheck',0,'EnableTriggerEvent',0,'TriggerMode',2,'TriggerLineOut',1,'ADCSWStartEnable',0,'SampleTime',-1,'SampleTimeCheck',1,'StatusPortEnable',0,'TLCFileName','rti120xadc_c1_adc')
  ADC_CLASS1_BL7 : rti1202lib_adc_class1/ADC_CLASS1_BL1  DSProperties=struct('RTI',struct('Version',uint32(1),'BlockType',struct('isSLSource',uint8(1),'isSLSink',uint8(1),'isHWSource',uint8(0),'isHWSink',uint8(1),'isSetup',uint8(0),'isInline',uint8(1),'isNonInline',uint8(0),'isInterrupt',uint8(0),'isChannelwise',uint8(1)),'IOBoardType',{{'DS120X','STD','ADCC1'}},'UnitType','ADC','Identifier','ADC','DialogType','ML','BlockSet','NONE','SlaveProcessor','NONE'))  RTIBlockInterface=struct('InputPortsActive',0,'InputPortsWidth',int32(1),'InputPortsDataType',{{'SS_BOOLEAN'}},'InputPortsName',{{'Continue'}},'OutputPortsActive',[1 0],'OutputPortsWidth',int32([1 1]),'OutputPortsDataType',{{'SS_DOUBLE','SS_INT16'}},'OutputPortsName',{{'ADC','Status'}},'DialogFcn','rti120xstdadcc1adcgui','SampleTime',{{-1}},'InitLevel',3,'IconTransparency','on','BlockDisplay',{{['ADC CL1\nChannel: 7'],'center'}},'BlockName',struct('Token',{{'ADC_CLASS1_BL1'}}))  RTIBlockParameters=struct('ReadMode',{{1,'OFF',[1 2]}},'ChannelNo',{{7,'OFF',[]}},'ConversionMode',{{1,'OFF',[1 2]}},'TriggerSource',{{1,'OFF',[1 2]}},'TriggerLineIn',{{1,'OFF',[1 16]}},'SampleMode',{{1,'OFF',[1 2]}},'BurstTriggerSource',{{1,'OFF',[1 2]}},'BurstTriggerLine',{{1,'OFF',[1 16]}},'ConvTriggerSource',{{3,'OFF',[1 3]}},'ConvTriggerLine',{{1,'OFF',[1 16]}},'ConvPeriod',{{'100e-6','OFF',[1e-6 1.34]}},'ConvPeriodCheck',{{0,'OFF',[]}},'BurstSize',{{'10','OFF',[]}},'BurstSizeCheck',{{0,'OFF',[]}},'DataSetOffset',{{'0','OFF',[]}},'DataSetOffsetCheck',{{0,'OFF',[]}},'DataSetLength',{{'1','OFF',[]}},'DataSetLengthCheck',{{0,'OFF',[]}},'EnableTriggerEvent',{{0,'OFF',[0 1]}},'TriggerMode',{{2,'OFF',[1 3]}},'TriggerLineOut',{{1,'OFF',[1 16]}},'ADCSWStartEnable',{{0,'OFF',[0 1]}},'SampleTime',{{'-1','OFF',[-1 inf]}},'SampleTimeCheck',{{1,'OFF',[]}},'StatusPortEnable',{{0,'OFF',[0 1]}},'TLCFileName',{{'rti120xadc_c1_adc','OFF',[]}})  RTISFcnParameters=struct('ReadMode','int16','ChannelNo','int16','ConversionMode','int16','TriggerSource','int16','TriggerLineIn','int16','SampleMode','int16','BurstTriggerSource','int16','BurstTriggerLine','int16','ConvTriggerSource','int16','ConvTriggerLine','int16','ConvPeriod','double','BurstSize','int16','DataSetOffset','int16','DataSetLength','int16','EnableTriggerEvent','int16','TriggerMode','int16','TriggerLineOut','int16','ADCSWStartEnable','int16','SampleTime','double','StatusPortEnable','int16','TLCFileName','char')  RTIBlockParaDefault=struct('ReadMode',1,'ChannelNo',1,'ConversionMode',1,'TriggerSource',1,'TriggerLineIn',1,'SampleMode',1,'BurstTriggerSource',1,'BurstTriggerLine',1,'ConvTriggerSource',3,'ConvTriggerLine',1,'ConvPeriod',0.0001,'ConvPeriodCheck',0,'BurstSize',10,'BurstSizeCheck',0,'DataSetOffset',0,'DataSetOffsetCheck',0,'DataSetLength',1,'DataSetLengthCheck',0,'EnableTriggerEvent',0,'TriggerMode',2,'TriggerLineOut',1,'ADCSWStartEnable',0,'SampleTime',-1,'SampleTimeCheck',1,'StatusPortEnable',0,'TLCFileName','rti120xadc_c1_adc')
  ADC_CLASS1_BL8 : rti1202lib_adc_class1/ADC_CLASS1_BL1  DSProperties=struct('RTI',struct('Version',uint32(1),'BlockType',struct('isSLSource',uint8(1),'isSLSink',uint8(1),'isHWSource',uint8(0),'isHWSink',uint8(1),'isSetup',uint8(0),'isInline',uint8(1),'isNonInline',uint8(0),'isInterrupt',uint8(0),'isChannelwise',uint8(1)),'IOBoardType',{{'DS120X','STD','ADCC1'}},'UnitType','ADC','Identifier','ADC','DialogType','ML','BlockSet','NONE','SlaveProcessor','NONE'))  RTIBlockInterface=struct('InputPortsActive',0,'InputPortsWidth',int32(1),'InputPortsDataType',{{'SS_BOOLEAN'}},'InputPortsName',{{'Continue'}},'OutputPortsActive',[1 0],'OutputPortsWidth',int32([1 1]),'OutputPortsDataType',{{'SS_DOUBLE','SS_INT16'}},'OutputPortsName',{{'ADC','Status'}},'DialogFcn','rti120xstdadcc1adcgui','SampleTime',{{-1}},'InitLevel',3,'IconTransparency','on','BlockDisplay',{{['ADC CL1\nChannel: 8'],'center'}},'BlockName',struct('Token',{{'ADC_CLASS1_BL1'}}))  RTIBlockParameters=struct('ReadMode',{{1,'OFF',[1 2]}},'ChannelNo',{{8,'OFF',[]}},'ConversionMode',{{1,'OFF',[1 2]}},'TriggerSource',{{1,'OFF',[1 2]}},'TriggerLineIn',{{1,'OFF',[1 16]}},'SampleMode',{{1,'OFF',[1 2]}},'BurstTriggerSource',{{1,'OFF',[1 2]}},'BurstTriggerLine',{{1,'OFF',[1 16]}},'ConvTriggerSource',{{3,'OFF',[1 3]}},'ConvTriggerLine',{{1,'OFF',[1 16]}},'ConvPeriod',{{'100e-6','OFF',[1e-6 1.34]}},'ConvPeriodCheck',{{0,'OFF',[]}},'BurstSize',{{'10','OFF',[]}},'BurstSizeCheck',{{0,'OFF',[]}},'DataSetOffset',{{'0','OFF',[]}},'DataSetOffsetCheck',{{0,'OFF',[]}},'DataSetLength',{{'1','OFF',[]}},'DataSetLengthCheck',{{0,'OFF',[]}},'EnableTriggerEvent',{{0,'OFF',[0 1]}},'TriggerMode',{{2,'OFF',[1 3]}},'TriggerLineOut',{{1,'OFF',[1 16]}},'ADCSWStartEnable',{{0,'OFF',[0 1]}},'SampleTime',{{'-1','OFF',[-1 inf]}},'SampleTimeCheck',{{1,'OFF',[]}},'StatusPortEnable',{{0,'OFF',[0 1]}},'TLCFileName',{{'rti120xadc_c1_adc','OFF',[]}})  RTISFcnParameters=struct('ReadMode','int16','ChannelNo','int16','ConversionMode','int16','TriggerSource','int16','TriggerLineIn','int16','SampleMode','int16','BurstTriggerSource','int16','BurstTriggerLine','int16','ConvTriggerSource','int16','ConvTriggerLine','int16','ConvPeriod','double','BurstSize','int16','DataSetOffset','int16','DataSetLength','int16','EnableTriggerEvent','int16','TriggerMode','int16','TriggerLineOut','int16','ADCSWStartEnable','int16','SampleTime','double','StatusPortEnable','int16','TLCFileName','char')  RTIBlockParaDefault=struct('ReadMode',1,'ChannelNo',1,'ConversionMode',1,'TriggerSource',1,'TriggerLineIn',1,'SampleMode',1,'BurstTriggerSource',1,'BurstTriggerLine',1,'ConvTriggerSource',3,'ConvTriggerLine',1,'ConvPeriod',0.0001,'ConvPeriodCheck',0,'BurstSize',10,'BurstSizeCheck',0,'DataSetOffset',0,'DataSetOffsetCheck',0,'DataSetLength',1,'DataSetLengthCheck',0,'EnableTriggerEvent',0,'TriggerMode',2,'TriggerLineOut',1,'ADCSWStartEnable',0,'SampleTime',-1,'SampleTimeCheck',1,'StatusPortEnable',0,'TLCFileName','rti120xadc_c1_adc')
  Compare To Zero3 : simulink/Logic and Bit Operations/Compare To Zero  relop=>=  OutDataTypeStr=boolean
  Constant1 : Constant  Value=-2*pi/3
  Constant2 : Constant  Value=2*pi/3
  Data Type Conversion : DataTypeConversion
  Gain1 : Gain  Gain=2*pi
  Integrator : Integrator
  MATLAB Function1 : MATLAB Function  TreatAsAtomicUnit=on
  Mux : Mux  Inputs=3
  Mux1 : Mux  Inputs=3
  Mux2 : Mux  Inputs=3
  PROC_SETUP_BL1 : rtiproclib/PROC_SETUP_BL1  DSProperties=struct('RTI',struct('Version',uint32(3),'BlockType',struct('isSLSource',uint8(0),'isSLSink',uint8(0),'isHWSource',uint8(0),'isHWSink',uint8(0),'isSetup',uint8(1),'isInline',uint8(1),'isNonInline',uint8(0),'isInterrupt',uint8(0),'isChannelwise',uint8(0)),'IOBoardType','DSPROC','UnitType','SETUP','Identifier','SETUP','DialogType','ML','BlockSet','NONE','SlaveProcessor',''))  RTIBlockInterface=struct('OutputPortsWidth',int32(0),'OutputPortsActive',0,'InitLevel',3,'DialogFcn','rtiprocsetupgui','BlockDisplay',{{['Processor Setup'],'auto'}},'IconTransparency','off','BlockName',struct('Token',{{'PROC_SETUP_BL1'}}))  RTIBlockParameters=struct('NumBoardsUsed',{{1,'OFF',[1 16]}},'ModelMode',{{1,'OFF',[]}},'IniFileList',{{struct('Fullname','','Filename','','Relname','','Assigned',0),'OFF',[]}},'SubsysList',{{struct('SharedAccess',1,'SetupBlockHandle',14964.005126953125,'SetupBlockName','FPGA_SETUP_BL1','SubsysName','4_step','SubsysHandle',12888.016723632813,'SubsysPath','/4_step','Assigned',1,'IniFilePath','D:\test1\test1_rtiFPGA/INI/4_step_7593219A2930B1.ini','IniFileName','4_step_7593219A2930B1','IniFileDate',739389.67724537035),'OFF',[]}},'AssignList',{{struct('BoardNumber',{1,2,3,4,5,6,7,8,9,10,11,12,13,14,15,16},'ModelType',{1,0,0,0,0,0,0,0,0,0,0,0,0,0,0,0},'ModelNo',{1,0,0,0,0,0,0,0,0,0,0,0,0,0,0,0},'ProgOption',{1,0,0,0,0,0,0,0,0,0,0,0,0,0,0,0},'IncludeBuild',{1,0,0,0,0,0,0,0,0,0,0,0,0,0,0,0},'IncludeProcAppl',{true,0,0,0,0,0,0,0,0,0,0,0,0,0,0,0}),'OFF',[]}},'ProcSetupHandles',{{-1,'OFF',[]}},'MaxNumBoards',{{16,'OFF',[]}},'ModelPath',{{'D:\MarcosGomez\test1','OFF',[]}},'FrameDir',{{[' '],'OFF',[]}},'TLCFileName',{{'rtiprocsetup','OFF',[]}},'IsNewBlock',{{0,'OFF',[]}},'NeedsCodeGen',{{1,'OFF',[]}})  RTISFcnParameters=struct('FrameDir','char','TLCFileName','char')  RTIBlockParaDefault=struct('NumBoardsUsed',1,'ModelMode',1,'IniFileList',struct('Fullname','','Filename','','Relname','','Assigned',''),'SubsysList',struct('SubsysName','','SubsysPath','','SubsysHandle','','SetupBlockHandle','','SetupBlockName','','Filename','','Relname','','IniFilePath','','IniFileName','','IniFileDate','','Assigned',''),'AssignList',struct('BoardNumber','','ModelType','','ModelNo','','ProgOption','','IncludeBuild','','IncludeProcAppl',''),'ProcSetupHandles',-1,'MaxNumBoards',16,'ModelPath',[' '],'FrameDir',[' '],'TLCFileName','rtiprocsetup','IsNewBlock',1,'NeedsCodeGen',0)
      settings: AttributesFormatString=FPGA-Build / Offline Simulation
  PROC_XDATA_WRITE_BL1 - cl : rtiproclib/PROC_XDATA_WRITE_BL1  DSProperties=struct('RTI',struct('Version',uint32(6),'BlockType',struct('isSLSource',uint8(0),'isSLSink',uint8(1),'isHWSource',uint8(0),'isHWSink',uint8(0),'isSetup',uint8(0),'isInline',uint8(1),'isNonInline',uint8(0),'isInterrupt',uint8(0),'isChannelwise',uint8(0)),'IOBoardType','DSPROC','UnitType','','Identifier','PHSWRITE','DialogType','ML','BlockSet','DSPROC','SlaveProcessor',''))  RTIBlockInterface=struct('InputPortsActive',true,'InputPortsWidth',{{'DYNAMICALLY_SIZED'}},'InputPortsDataType',{{'SS_DOUBLE'}},'InputPortsName',{{'Data'}},'InitLevel',3,'DialogFcn','rtiprocphswritegui','BlockDisplay',{{['Register Out 3\ncl\nGroup ID: 1 Board: 1'],'auto'}},'IconTransparency','on','BlockName',struct('Token',{{'PROC_XDATA_WRITE_BL1'}}))  RTIBlockParameters=struct('BoardNo',{{'1','OFF',[1 16]}},'ChannelNo',{{'3','OFF',[]}},'AccessTyp',{{'Register','OFF',[]}},'BinaryPoint',{{'0','OFF',[]}},'DataFormat',{{'unsigned','OFF',[]}},'BufferLength',{{'0','OFF',[]}},'GroupNo',{{'1','OFF',[]}},'MultiChAccess',{{'0','OFF',[]}},'InitOnly',{{'0','OFF',[]}},'InitValue',{{'0','OFF',[]}},'TLCFileName',{{'rtiprocphswrite','OFF',[]}},'ModelPortBlock',{{{struct('BlockId','','SignalId','')},'OFF',[]}})  RTISFcnParameters=struct('BoardNo','double','ChannelNo','double','GroupNo','double','AccessTyp','char','BinaryPoint','double','DataFormat','char','BufferLength','double','InitOnly','double','InitValue','double','TLCFileName','char')  RTIBlockParaDefault=struct('BoardNo','1','ChannelNo','0','AccessTyp','Register','BinaryPoint','10','DataFormat','signed','BufferLength','16','GroupNo','0','MultiChAccess','0','InitOnly','0','InitValue','0','TLCFileName','rtiprocphswrite','ModelPortBlock',{{struct('BlockId','','SignalId','','BusObject','')}})
  PROC_XDATA_WRITE_BL1 - dir : rtiproclib/PROC_XDATA_WRITE_BL1  DSProperties=struct('RTI',struct('Version',uint32(6),'BlockType',struct('isSLSource',uint8(0),'isSLSink',uint8(1),'isHWSource',uint8(0),'isHWSink',uint8(0),'isSetup',uint8(0),'isInline',uint8(1),'isNonInline',uint8(0),'isInterrupt',uint8(0),'isChannelwise',uint8(0)),'IOBoardType','DSPROC','UnitType','','Identifier','PHSWRITE','DialogType','ML','BlockSet','DSPROC','SlaveProcessor',''))  RTIBlockInterface=struct('InputPortsActive',true,'InputPortsWidth',{{'DYNAMICALLY_SIZED'}},'InputPortsDataType',{{'SS_DOUBLE'}},'InputPortsName',{{'Data'}},'InitLevel',3,'DialogFcn','rtiprocphswritegui','BlockDisplay',{{['Register Out 2\ndir \nGroup ID: 1 Board: 1'],'auto'}},'IconTransparency','on','BlockName',struct('Token',{{'PROC_XDATA_WRITE_BL1'}}))  RTIBlockParameters=struct('BoardNo',{{'1','OFF',[1 16]}},'ChannelNo',{{'2','OFF',[]}},'AccessTyp',{{'Register','OFF',[]}},'BinaryPoint',{{'0','OFF',[]}},'DataFormat',{{'unsigned','OFF',[]}},'BufferLength',{{'0','OFF',[]}},'GroupNo',{{'1','OFF',[]}},'MultiChAccess',{{'0','OFF',[]}},'InitOnly',{{'0','OFF',[]}},'InitValue',{{'0','OFF',[]}},'TLCFileName',{{'rtiprocphswrite','OFF',[]}},'ModelPortBlock',{{{struct('BlockId','','SignalId','')},'OFF',[]}})  RTISFcnParameters=struct('BoardNo','double','ChannelNo','double','GroupNo','double','AccessTyp','char','BinaryPoint','double','DataFormat','char','BufferLength','double','InitOnly','double','InitValue','double','TLCFileName','char')  RTIBlockParaDefault=struct('BoardNo','1','ChannelNo','0','AccessTyp','Register','BinaryPoint','10','DataFormat','signed','BufferLength','16','GroupNo','0','MultiChAccess','0','InitOnly','0','InitValue','0','TLCFileName','rtiprocphswrite','ModelPortBlock',{{struct('BlockId','','SignalId','','BusObject','')}})
  PROC_XDATA_WRITE_BL1 - lim : rtiproclib/PROC_XDATA_WRITE_BL1  DSProperties=struct('RTI',struct('Version',uint32(6),'BlockType',struct('isSLSource',uint8(0),'isSLSink',uint8(1),'isHWSource',uint8(0),'isHWSink',uint8(0),'isSetup',uint8(0),'isInline',uint8(1),'isNonInline',uint8(0),'isInterrupt',uint8(0),'isChannelwise',uint8(0)),'IOBoardType','DSPROC','UnitType','','Identifier','PHSWRITE','DialogType','ML','BlockSet','DSPROC','SlaveProcessor',''))  RTIBlockInterface=struct('InputPortsActive',true,'InputPortsWidth',{{'DYNAMICALLY_SIZED'}},'InputPortsDataType',{{'SS_DOUBLE'}},'InputPortsName',{{'Data'}},'InitLevel',3,'DialogFcn','rtiprocphswritegui','BlockDisplay',{{['Register Out 4\nlim\nGroup ID: 1 Board: 1'],'auto'}},'IconTransparency','on','BlockName',struct('Token',{{'PROC_XDATA_WRITE_BL1'}}))  RTIBlockParameters=struct('BoardNo',{{'1','OFF',[1 16]}},'ChannelNo',{{'4','OFF',[]}},'AccessTyp',{{'Register','OFF',[]}},'BinaryPoint',{{'0','OFF',[]}},'DataFormat',{{'unsigned','OFF',[]}},'BufferLength',{{'0','OFF',[]}},'GroupNo',{{'1','OFF',[]}},'MultiChAccess',{{'0','OFF',[]}},'InitOnly',{{'0','OFF',[]}},'InitValue',{{'0','OFF',[]}},'TLCFileName',{{'rtiprocphswrite','OFF',[]}},'ModelPortBlock',{{{struct('BlockId','','SignalId','')},'OFF',[]}})  RTISFcnParameters=struct('BoardNo','double','ChannelNo','double','GroupNo','double','AccessTyp','char','BinaryPoint','double','DataFormat','char','BufferLength','double','InitOnly','double','InitValue','double','TLCFileName','char')  RTIBlockParaDefault=struct('BoardNo','1','ChannelNo','0','AccessTyp','Register','BinaryPoint','10','DataFormat','signed','BufferLength','16','GroupNo','0','MultiChAccess','0','InitOnly','0','InitValue','0','TLCFileName','rtiprocphswrite','ModelPortBlock',{{struct('BlockId','','SignalId','','BusObject','')}})
  PROC_XDATA_WRITE_BL1 - v1 : rtiproclib/PROC_XDATA_WRITE_BL1  DSProperties=struct('RTI',struct('Version',uint32(6),'BlockType',struct('isSLSource',uint8(0),'isSLSink',uint8(1),'isHWSource',uint8(0),'isHWSink',uint8(0),'isSetup',uint8(0),'isInline',uint8(1),'isNonInline',uint8(0),'isInterrupt',uint8(0),'isChannelwise',uint8(0)),'IOBoardType','DSPROC','UnitType','','Identifier','PHSWRITE','DialogType','ML','BlockSet','DSPROC','SlaveProcessor',''))  RTIBlockInterface=struct('InputPortsActive',true,'InputPortsWidth',{{'DYNAMICALLY_SIZED'}},'InputPortsDataType',{{'SS_DOUBLE'}},'InputPortsName',{{'Data'}},'InitLevel',3,'DialogFcn','rtiprocphswritegui','BlockDisplay',{{['Register Out 1\nv \nGroup ID: 1 Board: 1'],'auto'}},'IconTransparency','on','BlockName',struct('Token',{{'PROC_XDATA_WRITE_BL1'}}))  RTIBlockParameters=struct('BoardNo',{{'1','OFF',[1 16]}},'ChannelNo',{{'1','OFF',[]}},'AccessTyp',{{'Register','OFF',[]}},'BinaryPoint',{{'0','OFF',[]}},'DataFormat',{{'unsigned','OFF',[]}},'BufferLength',{{'0','OFF',[]}},'GroupNo',{{'1','OFF',[]}},'MultiChAccess',{{'0','OFF',[]}},'InitOnly',{{'0','OFF',[]}},'InitValue',{{'0','OFF',[]}},'TLCFileName',{{'rtiprocphswrite','OFF',[]}},'ModelPortBlock',{{{struct('BlockId','','SignalId','')},'OFF',[]}})  RTISFcnParameters=struct('BoardNo','double','ChannelNo','double','GroupNo','double','AccessTyp','char','BinaryPoint','double','DataFormat','char','BufferLength','double','InitOnly','double','InitValue','double','TLCFileName','char')  RTIBlockParaDefault=struct('BoardNo','1','ChannelNo','0','AccessTyp','Register','BinaryPoint','10','DataFormat','signed','BufferLength','16','GroupNo','0','MultiChAccess','0','InitOnly','0','InitValue','0','TLCFileName','rtiprocphswrite','ModelPortBlock',{{struct('BlockId','','SignalId','','BusObject','')}})
  Product : Product
  Product1 : Product
  RTI Data : Subsystem  Tag=struct('RTIDataServer',struct('RTIDataServerVs','2','RTIModelDescription','struct(''main'',''test1'',''sub'','''',''isMp'',0)'))  LoadFcn="if exist('rtidc'), try,  rtidc('DataHostBlockClbLoad', gcbh); catch, disp(['Warning: ''LoadFcn'' for RTI Data block failed: ' lasterr]); end, end,"  mask(RTI_DATA_HOST){}
      mask help:
      | RTI Data Block.
      | This block is used by RTI to store internal model-dependent data.
      | Please keep this block on the root level of the model. Deleting this block will result in data loss.
      |
      | NEVER DELETE OR COPY THIS BLOCK!
      settings: CopyFcn="if exist('rtidc'), try,  rtidc('DataHostBlockClbCopy', gcbh); catch, disp(['Warning: ''CopyFcn'' for RTI Data block failed: ' lasterr]); end, end,"  DeleteFcn="if exist('rtidc'), try,  rtidc('DataHostBlockClbDelete', gcbh); catch, disp(['Warning: ''DeleteFcn'' for RTI Data block failed: ' lasterr]); end, end,"  ModelCloseFcn="if exist('rtidc'), try,  rtidc('DataHostBlockClbModelClose', gcbh); catch, disp(['Warning: ''ModelCloseFcn'' for RTI Data block failed: ' lasterr]); end, end,"  PreSaveFcn="if exist('rtidc'), try,  rtidc('DataHostBlockClbPreSave', gcbh); catch, disp(['Warning: ''PreSaveFcn'' for RTI Data block failed: ' lasterr]); end, end,"  PostSaveFcn="if exist('rtidc'), try,  rtidc('DataHostBlockClbPostSave', gcbh); catch, disp(['Warning: ''PostSaveFcn'' for RTI Data block failed: ' lasterr]); end, end,"  NameChangeFcn="if exist('rtidc'), try,  rtidc('DataHostBlockClbNameChange', gcbh); catch, disp(['Warning: ''NameChangeFcn'' for RTI Data block failed: ' lasterr]); end, end,"
      mask Help:
      | RTI Data Block.
      | This block is used by RTI to store internal model-dependent data.
      | Please keep this block on the root level of the model. Deleting this block will result in data loss.
      | 
      | NEVER DELETE OR COPY THIS BLOCK!
      mask Display:
      | text(0.5, 0.5, 'RTI Data', 'HorizontalAlignment', 'center');
      | plot([1 0]);
  Relational Operator : RelationalOperator  OutDataTypeStr=boolean  RndMeth=Simplest
  Sin : Trigonometry
  Subsystem : Subsystem
  Sum7 : Sum  Inputs=++|
  Sum8 : Sum  Inputs=++|
  clamp_threshold : Constant  Value=clamp_threshold
  dir : Constant
  estado : Constant
  freq : Constant  Value=60
  ia : Sum  Inputs=|++
  ib : Sum  Inputs=|++
  ic : Sum  Inputs=|++
  ioa_fixed_gain : Gain  Gain=io_fixed_gain
  ioa_gain : Gain  Gain=ioa_gain
  ioa_offset : Constant  Value=ioa_offset
  ioa_sonda : Gain  Gain=io_sonda_gain
  iob_fixed_gain : Gain  Gain=io_fixed_gain
  iob_gain : Gain  Gain=iob_gain
  iob_offset : Constant  Value=iob_offset
  ioc_fixed_gain : Gain  Gain=io_fixed_gain
  ioc_gain : Gain  Gain=ioc_gain
  ioc_offset : Constant  Value=ioc_offset
  iref_amplitude : Gain
  limit : Constant  Value=5
  limit1 : Constant  Value=Ts
  v_clamp : Sum  Inputs=|++
  vclamp_gain : Gain  Gain=vclamp_gain
  vclamp_offset : Constant  Value=vclamp_offset
  via : Sum  Inputs=|++
  via_fixed_gain : Gain  Gain=vi_fixed_gain
  via_gain : Gain  Gain=via_gain
  via_offset : Constant  Value=via_offset
  via_sonda : Gain  Gain=vi_sonda_gain
  vib : Sum  Inputs=|++
  vib_fixed_gain : Gain  Gain=vi_fixed_gain
  vib_gain : Gain  Gain=vib_gain
  vib_offset : Constant  Value=vib_offset
  vic : Sum  Inputs=|++
  vic_fixed_gain : Gain  Gain=vi_fixed_gain
  vic_gain : Gain  Gain=vic_gain
  vic_offset : Constant  Value=vic_offset
  wires:
  MATLAB Function1/1(y) -> PROC_XDATA_WRITE_BL1 - dir/1
  Relational Operator/1 -> Data Type Conversion/1  "clamp_act"
  ADC_CLASS1_BL1/1 -> ioa_fixed_gain/1
  iref_amplitude/1 -> Subsystem/1(iref)  "iref"
  clamp_threshold/1 -> Product1/1, Product1/2  "clamp_threshold"
  ioa_offset/1 -> ia/2
  ADC_CLASS1_BL2/1 -> iob_fixed_gain/1
  iob_offset/1 -> ib/2
  ADC_CLASS1_BL3/1 -> ioc_fixed_gain/1
  ioc_offset/1 -> ic/2
  ib/1 -> iob_gain/1
  ia/1 -> ioa_gain/1
  via/1 -> via_gain/1
  vib/1 -> vib_gain/1
  ADC_CLASS1_BL6/1 -> vic_fixed_gain/1
  ADC_CLASS1_BL4/1 -> via_fixed_gain/1
  vic_offset/1 -> vic/2
  vic/1 -> vic_gain/1
  via_offset/1 -> via/2
  ADC_CLASS1_BL5/1 -> vib_fixed_gain/1
  vib_offset/1 -> vib/2
  [ia] -> Mux/1
  ic/1 -> ioc_gain/1
  [ib] -> Mux/2
  [ic] -> Mux/3
  vclamp_offset/1 -> v_clamp/2
  ADC_CLASS1_BL7/1 -> vclamp_gain/1
  v_clamp/1 -> Product/1, Product/2  "v_clamp"
  Mux/1 -> Compare To Zero3/1, Subsystem/2(io)  "io"
  Mux1/1 -> Subsystem/3(vi)  "vi"
  Subsystem/1(s) -> PROC_XDATA_WRITE_BL1 - v1/1
  freq/1 -> Gain1/1
  Integrator/1 -> Mux2/1, Sum7/1, Sum8/1  "wt"
  Sin/1 -> iref_amplitude/1  "iref"
  Constant2/1 -> Sum8/2
  Constant1/1 -> Sum7/2
  Sum7/1 -> Mux2/2
  Sum8/1 -> Mux2/3
  Mux2/1 -> Sin/1
  dir/1 -> ?
  limit/1 -> PROC_XDATA_WRITE_BL1 - lim/1
  Product/1 -> Relational Operator/1
  Product1/1 -> Relational Operator/2
  vclamp_gain/1 -> v_clamp/1
  via_fixed_gain/1 -> via/1
  vib_fixed_gain/1 -> vib/1
  vic_fixed_gain/1 -> vic/1
  ioc_fixed_gain/1 -> ic/1
  iob_fixed_gain/1 -> ib/1
  ioa_fixed_gain/1 -> ia/1
  Compare To Zero3/1 -> MATLAB Function1/1(u)
  vic_gain/1 -> Mux1/3
  vib_gain/1 -> Mux1/2
  via_gain/1 -> Mux1/1
  ioc_gain/1 -> [ic]  "ioc"
  iob_gain/1 -> [ib]  "iob"
  ioa_gain/1 -> [ia]  "ioc"
  ADC_CLASS1_BL8/1 -> via_sonda/1
  ADC_CLASS1_BL11/1 -> ioa_sonda/1
  limit1/1 -> Subsystem/4(T)
  Gain1/1 -> Integrator/1
  Data Type Conversion/1 -> PROC_XDATA_WRITE_BL1 - cl/1
  estado/1 -> ?
